simulink model "Car2WithArduinoPins"  (R2024a)
settings: Solver=VariableStepAuto  StartTime=0.0  StopTime=10.0  RelTol=1e-3
libraries: arduinolib x2
settings Model: Creator=thipp  LastModifiedBy=thipp

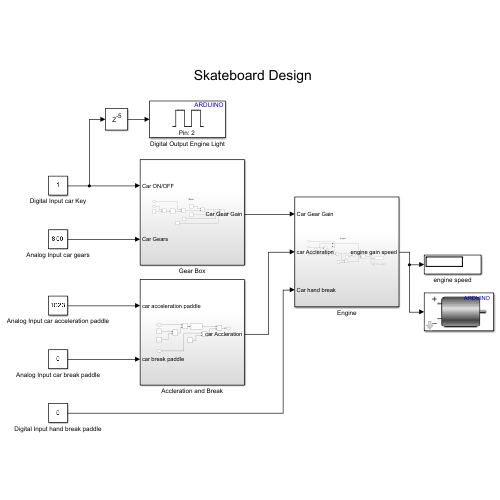
[thumbnail: Simulink's stored preview of the top-level diagram]
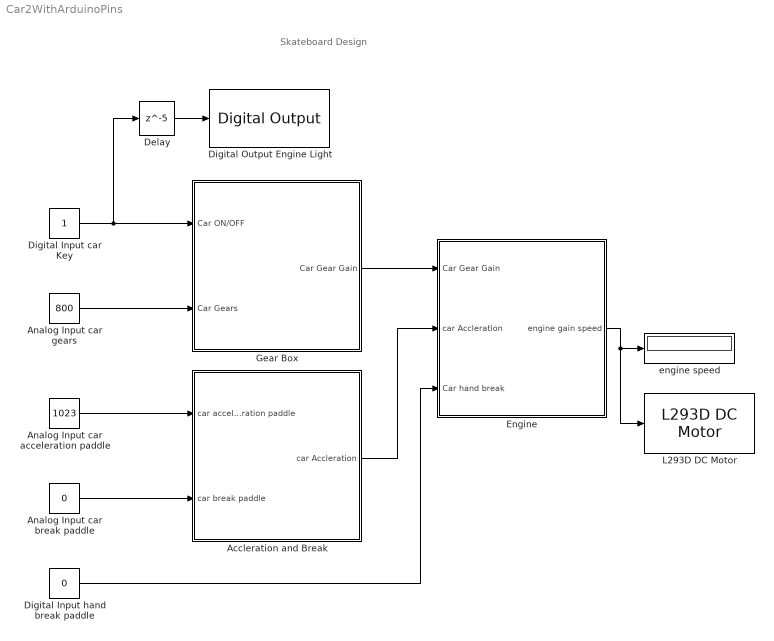
== system Car2WithArduinoPins ==
  note: Skateboard Design
  Accleration and Break : Subsystem
  Analog Input car acceleration paddle : Constant  Value=1023
  Analog Input car break paddle : Constant  Value=0
  Analog Input car gears : Constant  Value=800
  Delay : Delay  DelayLength=5
  Digital Input car Key : Constant
  Digital Input hand break paddle : Constant  Value=0
  Digital Output Engine Light : arduinolib/Digital Output  pinNumber=2  Direction=output  blockPlatform=arduino
  Engine : Subsystem
  Gear Box : Subsystem
  L293D DC Motor : arduinolib/L293D DC Motor  EnablePin=11  InputAPin=10  InputBPin=9
  engine speed : Display
  wires:
  Digital Input car Key/1 -> Delay/1, Gear Box/1(Car ON/OFF)
  Analog Input car acceleration paddle/1 -> Accleration and Break/1(car acceleration paddle)
  Analog Input car break paddle/1 -> Accleration and Break/2(car break paddle)
  Analog Input car gears/1 -> Gear Box/2(Car Gears)
  Engine/1(engine gain speed) -> engine speed/1, L293D DC Motor/1
  Gear Box/1(Car Gear Gain) -> Engine/1(Car Gear Gain)
  Accleration and Break/1(car Accleration) -> Engine/2(car Accleration)
  Digital Input hand break paddle/1 -> Engine/3("Car hand break ")
  Delay/1 -> Digital Output Engine Light/1

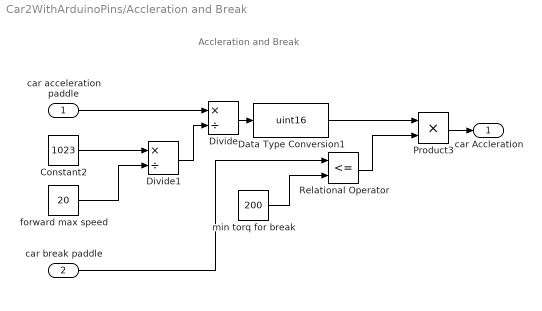
== system Car2WithArduinoPins/Accleration and Break ==
  note: Accleration and Break
  car acceleration paddle : Inport
  car break paddle : Inport  Port=2
  Constant2 : Constant  Value=1023
  Data Type Conversion1 : DataTypeConversion  OutDataTypeStr=uint16  SaturateOnIntegerOverflow=off  RndMeth=Floor
  Divide : Product  Inputs=*/  RndMeth=Zero  SaturateOnIntegerOverflow=on
  Divide1 : Product  Inputs=*/  RndMeth=Zero  SaturateOnIntegerOverflow=on
  Product3 : Product
  Relational Operator : RelationalOperator  Operator=<=  OutDataTypeStr=boolean  RndMeth=Simplest  InputSameDT=off
  forward max speed : Constant  Value=20
  min torq for break : Constant  Value=200
  car Accleration : Outport
  wires:
  min torq for break/1 -> Relational Operator/2
  Divide/1 -> Data Type Conversion1/1
  forward max speed/1 -> Divide1/2
  car break paddle/1 -> Relational Operator/1
  Data Type Conversion1/1 -> Product3/1
  Constant2/1 -> Divide1/1
  Divide1/1 -> Divide/2
  Relational Operator/1 -> Product3/2
  car acceleration paddle/1 -> Divide/1
  Product3/1 -> car Accleration/1

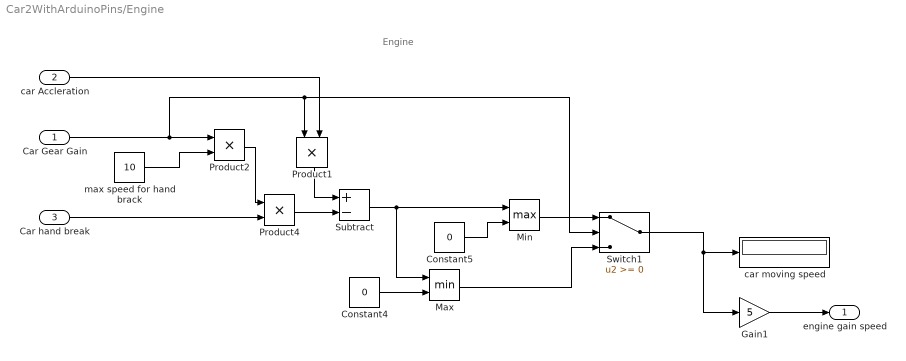
== system Car2WithArduinoPins/Engine ==
  note: Engine
  Car Gear Gain : Inport
  car Accleration : Inport  Port=2
  "Car hand break " : Inport  Port=3
  Constant4 : Constant  Value=0
  Constant5 : Constant  Value=0
  Gain1 : Gain  Gain=5
  Max : MinMax  Inputs=2
  Min : MinMax  Function=max  Inputs=2
  Product1 : Product
  Product2 : Product
  Product4 : Product
  Subtract : Sum  Inputs=+-
  Switch1 : Switch  SaturateOnIntegerOverflow=off  InputSameDT=off
  car moving speed : Display
  max speed for hand brack : Constant  Value=10
  engine gain speed : Outport
  wires:
  Subtract/1 -> Min/1, Max/1
  Switch1/1 -> Gain1/1, car moving speed/1
  Product2/1 -> Product4/1
  Product1/1 -> Subtract/1
  Product4/1 -> Subtract/2
  Constant5/1 -> Min/2
  max speed for hand brack/1 -> Product2/2
  Car Gear Gain/1 -> Product1/1, Switch1/2, Product2/1
  Max/1 -> Switch1/3
  Min/1 -> Switch1/1
  Constant4/1 -> Max/2
  car Accleration/1 -> Product1/2
  "Car hand break "/1 -> Product4/2
  Gain1/1 -> engine gain speed/1

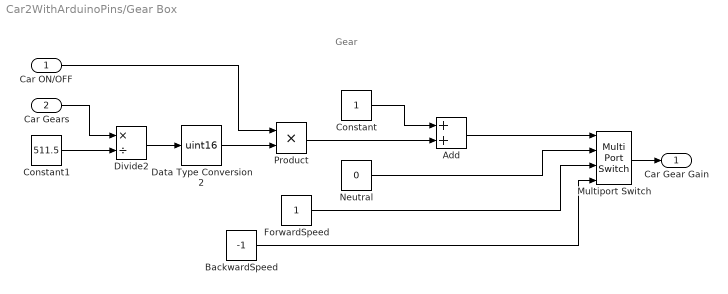
== system Car2WithArduinoPins/Gear Box ==
  note: Gear
  Car ON/OFF : Inport
  Car Gears : Inport  Port=2
  Add : Sum
  BackwardSpeed : Constant  Value=-1
  Constant : Constant
  Constant1 : Constant  Value=511.5
  Data Type Conversion2 : DataTypeConversion  OutDataTypeStr=uint16  RndMeth=Nearest  SaturateOnIntegerOverflow=off
  Divide2 : Product  Inputs=*/  RndMeth=Zero  SaturateOnIntegerOverflow=on
  ForwardSpeed : Constant
  Multiport Switch : MultiPortSwitch  SaturateOnIntegerOverflow=off  InputSameDT=off
  Neutral : Constant  Value=0
  Product : Product
  Car Gear Gain : Outport
  wires:
  Add/1 -> Multiport Switch/1
  Neutral/1 -> Multiport Switch/2
  Constant1/1 -> Divide2/2
  Product/1 -> Add/2
  BackwardSpeed/1 -> Multiport Switch/4
  Data Type Conversion2/1 -> Product/2
  ForwardSpeed/1 -> Multiport Switch/3
  Divide2/1 -> Data Type Conversion2/1
  Constant/1 -> Add/1
  Car Gears/1 -> Divide2/1
  Multiport Switch/1 -> Car Gear Gain/1
  Car ON/OFF/1 -> Product/1
